simulink model "PID_PMSM_Version_final"  (R2022b)
settings: Solver=VariableStepAuto  StartTime=0.0  StopTime=6  RelTol=1e-3
InitFcn:
  | %% PMSM parameter initialization
  | % switching freq, sample time
  | Ts = 5e-6;          % Fundamental sample time
  | Fsw = 5e3;          % Switching frequency (Hz)
  | Tsw =  1/Fsw ;      %1/Fsw ; Time Switching
  | Tsc = 5e-6  ;       %1/fc;  % Control loop sample time
  | fc = 1/Tsc;         % Control loop frequency (Hz)
  | % ================================================
  | 
  | % PMSM parameters
  | Ld = 0.006365;          % Stator inductance
  | Lq = 0.006365 ;
  | Rs = 1.6;               % Stator Resistance
  | Lambda_m = 0.1852;      % Permanent Flux linkage
  | Polepairs = 4; N = 4;   % Number of pole pairs
  | J = 0.0001854;          % Moment of inertia
  | B = 5.39e-5;            % Viscous coefficient
  | 
  | Vnorm = 300;            % Vdc voltage (DC-bus)
  | Vbat = 350 ;           % Battery voltage (supply the inverter)
undefined symbols (not defined in the file or in its folder): sigbuilder_block
libraries: spsIGBTDiodeLib x6, slpidlib x3, spsDCVoltageSourceLib x1, spsGroundLib x1, spsPermanentMagnetSynchronousMachineLib x1, spsThreePhaseVIMeasurementLib x1, spsCurrentMeasurementLib x1, spsVoltageMeasurementLib x1, eeTransforms x1, simulink_extras x1, spspowerguiLib x1
settings Model: Creator=M. Yahia  LastModifiedBy=muham

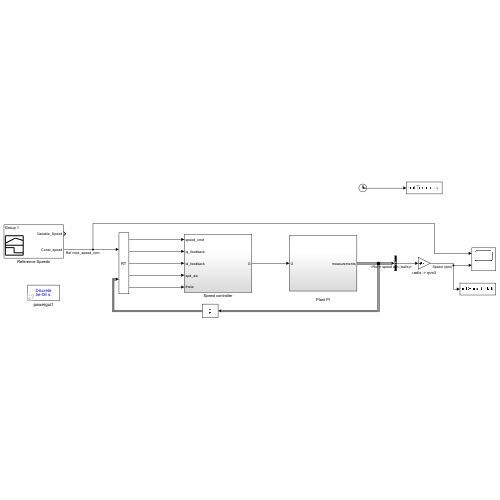
[thumbnail: Simulink's stored preview of the top-level diagram]
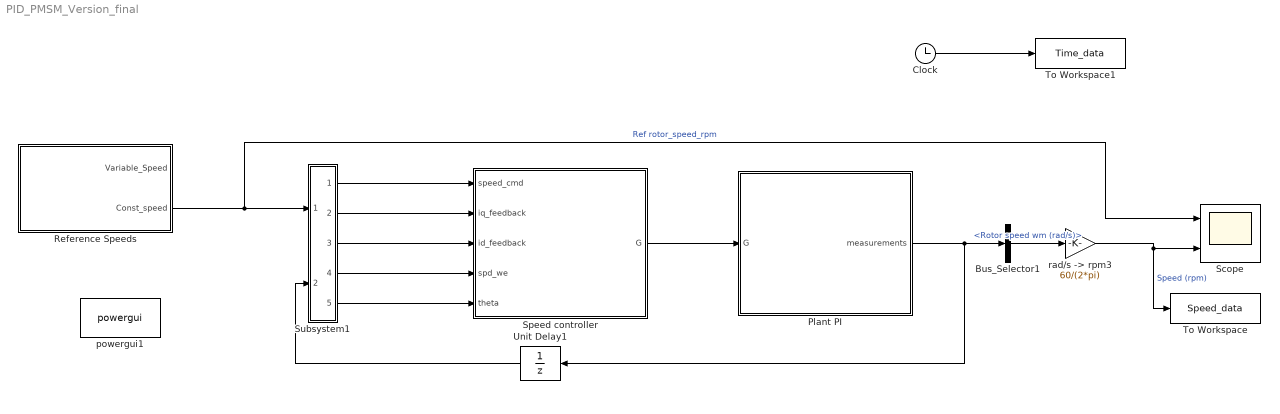
== system PID_PMSM_Version_final ==
  " Plant PI" : Subsystem
  Bus_Selector1 : BusSelector  OutputSignals=Rotor speed wm (rad/s)
  Clock : Clock
  Reference Speeds : Subsystem  Tag=STV Subsys  LoadFcn=sigbuilder_block('load');  StartFcn=sigbuilder_block('start');  StopFcn=sigbuilder_block('stop');  ClipboardFcn=sigbuilder_block('clipboard');  mask(Sigbuilder block){tuvar=[0:10]}
      mask help: Simulink:masks:SigbuilderBlock_MD
      mask init:
      | if ~strcmp(get_param(bdroot(gcbh),'SimulationStatus'),'stopped') tuvar = sigbuilder_block('maskInit'); end
      settings: CopyFcn=sigbuilder_block('copy');  DeleteFcn=sigbuilder_block('delete');  ModelCloseFcn=sigbuilder_block('modelClose');  PreSaveFcn=sigbuilder_block('preSave');  PauseFcn=sigbuilder_block('pause');  ContinueFcn=sigbuilder_block('continue');  NameChangeFcn=sigbuilder_block('namechange');  OpenFcn=sigbuilder_block('open',[34.8 97.5 688.2 385.125 ]);  CloseFcn=sigbuilder_block('close');
      mask Display: plot(0, 0, 100, 100,[2, 2, 32, 32, 2], [68, 8, 8, 68, 68],[32, 2], [38, 38], [32, 19, 2],[53, 60, 44], [32, 17, 17, 2],[16, 16, 31, 31]);txt = getActiveGroup(gcbh);text(2, 100, txt,'verticalAlignment', 'top');
  Scope : Scope  NumInputPorts=2
  Speed controller : Subsystem
  Subsystem1 : Subsystem
      mask Display: fprintf('RT')
  To Workspace : ToWorkspace  VariableName=Speed_data  SaveFormat=Timeseries  SampleTime=-1
  To Workspace1 : ToWorkspace  VariableName=Time_data  SaveFormat=Timeseries  SampleTime=-1
  Unit Delay1 : UnitDelay  SampleTime=-1  HasFrameUpgradeWarning=on
  powergui1 : spspowerguiLib/powergui  SimulationMode=Discrete  SampleTime=Ts  frequency=60  Iterations=50  frequencyindice=0  Pbase=100e6  ErrMax=1e-4  UnitsV=kV  UnitsW=MW  buscounter=0  FunctionMessages=off  echomessages=off  EnableUseOfTLC=off  CurrentSourceSwitches=off  DisableSnubberDevices=off  DisableRonSwitches=off  DisableVfSwitches=off  DisplayEquations=off  AutomaticDiscreteSolvers=off  SolverType=Tustin/Backward Euler (TBE)  Interpol=off  ExternalGateDelay=off  methode=off  Ts=100  x0status=blocks  SPID=on  SwTol=0  HookPort=off  NonlinearTolerance=1e-4  nMaxIteration=100  ContinueOnMaxIteration=off  RestoreLinks=warning  ResistiveCurrentMeasurement=off  Frange=[0:2:500]  Ylog=off  Xlog=on  ShowGrid=off  save=off  variable=ZData  structure=0  ZoomFFT=on  StartTime=0.0  cycles=1  DisplayStyle=1  fundamental=60  FreqAxis=off  MaxFrequency=1000  frequencyindicesteady=1  RmsSteady=1  display=off
  "rad/s -> rpm3" : Gain  Gain=60/(2*pi)
  wires:
  Unit Delay1/1 -> Subsystem1/2(PMSM_Measurements)
  Bus_Selector1/1 -> "rad/s -> rpm3"/1  "<Rotor speed wm (rad/s)>"
  Subsystem1/3(Out3) -> Speed controller/3(id_feedback)
  Speed controller/1(G) -> " Plant PI"/1(G)
  " Plant PI"/1(measurements) -> Bus_Selector1/1, Unit Delay1/1
  Subsystem1/4(Out1) -> Speed controller/4(spd_we)
  Subsystem1/2(Out2) -> Speed controller/2(iq_feedback)
  Subsystem1/5(Out4) -> Speed controller/5(theta)
  Subsystem1/1(Out6) -> Speed controller/1(speed_cmd)
  "rad/s -> rpm3"/1 -> To Workspace/1, Scope/2  "Speed (rpm)"
  Clock/1 -> To Workspace1/1
  Reference Speeds/2(Const_speed) -> Scope/1, Subsystem1/1(speed_cmd)  "Ref rotor_speed_rpm"

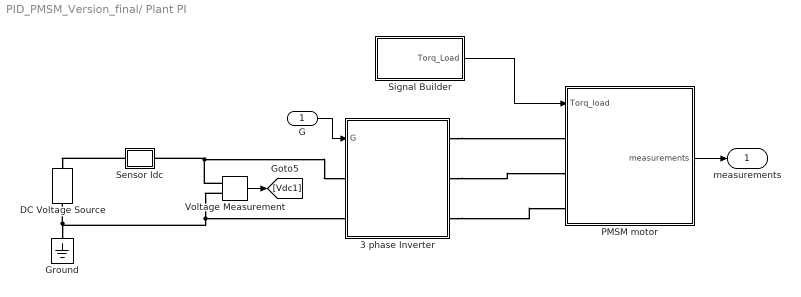
== system PID_PMSM_Version_final/ Plant PI ==
  G : Inport
  3 phase Inverter : Subsystem
  DC Voltage Source : spsDCVoltageSourceLib/DC Voltage Source  Amplitude=Vbat  Measurements=None
  Ground : spsGroundLib/Ground  LConnTagsString=a
  PMSM motor : Subsystem
  Sensor Idc : Subsystem
      mask Display: disp('Idc')
  Signal Builder : Subsystem  Tag=STV Subsys  LoadFcn=sigbuilder_block('load');  StartFcn=sigbuilder_block('start');  StopFcn=sigbuilder_block('stop');  ClipboardFcn=sigbuilder_block('clipboard');  mask(Sigbuilder block){tuvar=[0:10]}
      mask help: Simulink:masks:SigbuilderBlock_MD
      mask init:
      | if ~strcmp(get_param(bdroot(gcbh),'SimulationStatus'),'stopped') tuvar = sigbuilder_block('maskInit'); end
      settings: CopyFcn=sigbuilder_block('copy');  DeleteFcn=sigbuilder_block('delete');  ModelCloseFcn=sigbuilder_block('modelClose');  PreSaveFcn=sigbuilder_block('preSave');  PauseFcn=sigbuilder_block('pause');  ContinueFcn=sigbuilder_block('continue');  NameChangeFcn=sigbuilder_block('namechange');  OpenFcn=sigbuilder_block('open',[354.375 129 543.75 350.625 ]);  CloseFcn=sigbuilder_block('close');
      mask Display: plot(0, 0, 100, 100,[2, 2, 32, 32, 2], [68, 8, 8, 68, 68],[32, 2], [38, 38], [32, 19, 2],[53, 60, 44], [32, 17, 17, 2],[16, 16, 31, 31]);txt = getActiveGroup(gcbh);text(2, 100, txt,'verticalAlignment', 'top');
  Voltage Measurement : spsVoltageMeasurementLib/Voltage Measurement  PhasorSimulation=off  OutputType=Complex  PSBequivalent=0
  measurements : Outport
  wires:
  G/1 -> 3 phase Inverter/1(G)
  Voltage Measurement/1 -> [Vdc1]
  PMSM motor/1(measurements) -> measurements/1
  Signal Builder/1(Torq_Load) -> PMSM motor/1(Torq_load)
  connections:
  Voltage Measurement/LConn2 -- Ground/LConn1 -- DC Voltage Source/LConn1 -- 3 phase Inverter/LConn2
  Voltage Measurement/LConn1 -- Sensor Idc/RConn1 -- 3 phase Inverter/LConn1
  Sensor Idc/LConn1 -- DC Voltage Source/RConn1
  3 phase Inverter/RConn1 -- PMSM motor/LConn1
  3 phase Inverter/RConn2 -- PMSM motor/LConn2
  3 phase Inverter/RConn3 -- PMSM motor/LConn3

== system PID_PMSM_Version_final/Reference Speeds ==
  Demux : Demux  Tag=STV Demux  Outputs=2
      settings: DisplayOption=none
  FromWs : FromWorkspace  Tag=STV FromWs  VariableName=tuvar
      SigBuilderData=|
      | common.afterFinalStr = 'Extrapolate'
      | common.sampleTime = 0
      | dataSet.timeRange = [0 6]
      | dataSet.name = 'Group 1'
      | sbobj.Groups.Name = 'Group 1'
      | sbobj.Groups.Signals(1).Name = 'Variable_Speed'
      | sbobj.Groups.Signals(1).XData = [0 0.2 0.5 0.7 0.8 1.2 1.5 2.2 2.2 2.8 3 3.5 4 4.5 4.5 5.5 6]
      | sbobj.Groups.Signals(1).YData = [40 40 500 200 1000 1000 450 1500 2000 2000 600 600 2000 2000 1000 200 20]
      | sbobj.Groups.Signals(2).Name = 'Const_speed'
      | sbobj.Groups.Signals(2).XData = [0 6]
      | sbobj.Groups.Signals(2).YData = [1000 1000]
      | sbobj.Groups.TimeRange = [0 6]
  Variable_Speed : Outport  Tag=STV Outport  VectorParamsAs1DForOutWhenUnconnected=off
  Const_speed : Outport  Tag=STV Outport  Port=2
  wires:
  Demux/1 -> Variable_Speed/1
  FromWs/1 -> Demux/1
  Demux/2 -> Const_speed/1

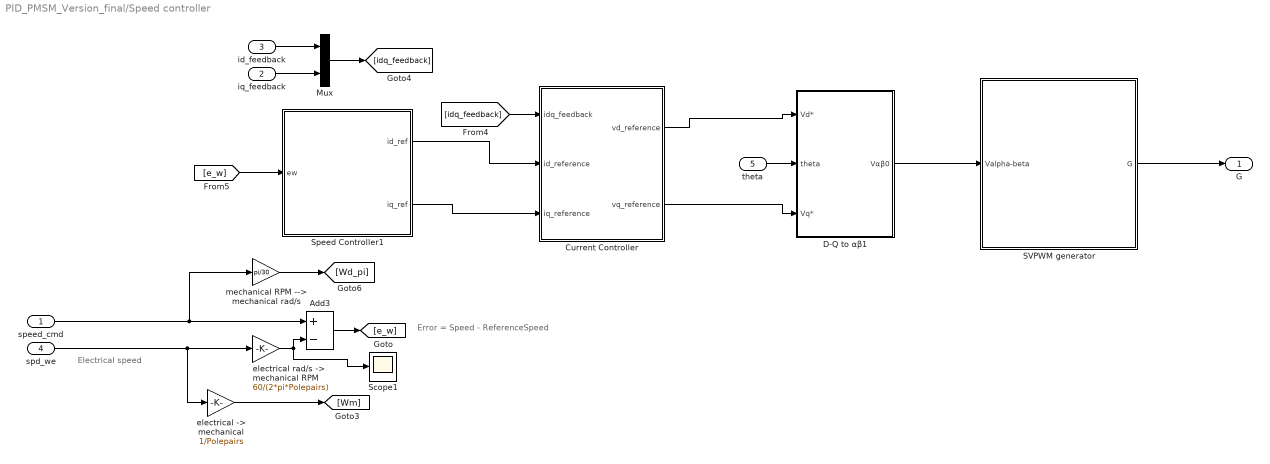
== system PID_PMSM_Version_final/Speed controller ==
  note: Error = Speed - ReferenceSpeed
  note: Electrical speed
  speed_cmd : Inport
  iq_feedback : Inport  Port=2  SampleTime=1e-4
  id_feedback : Inport  Port=3  SampleTime=1e-4
  spd_we : Inport  Port=4
  theta : Inport  Port=5  SampleTime=1e-4
  Add3 : Sum  Inputs=+-
  Current Controller : Subsystem
  D-Q to αβ1 : Subsystem
  Mux : Mux  Inputs=2
  SVPWM generator : Subsystem
  Scope1 : Scope
  Speed Controller1 : Subsystem
  "electrical -> mechanical" : Gain  Gain=1/Polepairs
  "electrical rad/s -> mechanical RPM" : Gain  Gain=60/(2*pi*Polepairs)
  "mechanical RPM --> mechanical rad/s " : Gain  Gain=pi/30
  G : Outport
  wires:
  Speed Controller1/2(iq_ref) -> Current Controller/3(iq_reference)
  Speed Controller1/1(id_ref) -> Current Controller/2(id_reference)
  id_feedback/1 -> Mux/1
  iq_feedback/1 -> Mux/2
  theta/1 -> D-Q to αβ1/2(theta)
  Add3/1 -> [e_w]
  "electrical -> mechanical"/1 -> [Wm]
  spd_we/1 -> "electrical -> mechanical"/1, "electrical rad/s -> mechanical RPM"/1
  "electrical rad/s -> mechanical RPM"/1 -> Scope1/1, Add3/2
  speed_cmd/1 -> "mechanical RPM --> mechanical rad/s "/1, Add3/1
  "mechanical RPM --> mechanical rad/s "/1 -> [Wd_pi]
  Mux/1 -> [idq_feedback]
  [idq_feedback] -> Current Controller/1(idq_feedback)
  [e_w] -> Speed Controller1/1(ew)
  Current Controller/1(vd_reference) -> D-Q to αβ1/1(Vd*)
  Current Controller/2(vq_reference) -> D-Q to αβ1/3(Vq*)
  SVPWM generator/1(G) -> G/1
  D-Q to αβ1/1("Vαβ0 ") -> SVPWM generator/1(Valpha-beta)

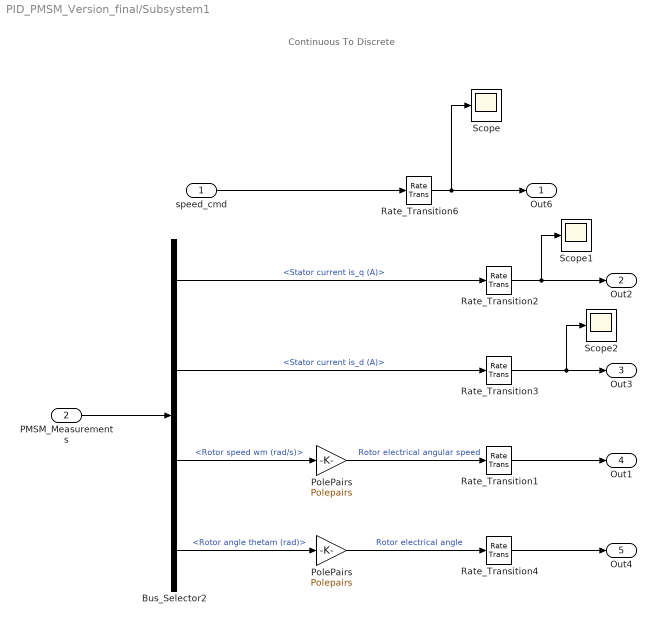
== system PID_PMSM_Version_final/Subsystem1 ==
  note: Continuous To Discrete
  speed_cmd : Inport
  PMSM_Measurements : Inport  Port=2
  Bus_Selector2 : BusSelector  OutputSignals=Stator current is_q (A),Stator current is_d (A),Rotor speed wm (rad/s),Rotor angle thetam (rad)
  PolePairs : Gain  Gain=Polepairs
  "PolePairs " : Gain  Gain=Polepairs
  Rate_Transition{1..4,6} (5 alike) : RateTransition  Integrity=off  Deterministic=off
  Scope : Scope
  Scope1 : Scope
  Scope2 : Scope
  Out6 : Outport  VectorParamsAs1DForOutWhenUnconnected=off
  Out2 : Outport  Port=2  VectorParamsAs1DForOutWhenUnconnected=off
  Out3 : Outport  Port=3  VectorParamsAs1DForOutWhenUnconnected=off
  Out1 : Outport  Port=4  VectorParamsAs1DForOutWhenUnconnected=off
  Out4 : Outport  Port=5  VectorParamsAs1DForOutWhenUnconnected=off
  wires:
  Rate_Transition4/1 -> Out4/1
  Bus_Selector2/2 -> Rate_Transition3/1  "<Stator current is_d (A)>"
  speed_cmd/1 -> Rate_Transition6/1
  Bus_Selector2/1 -> Rate_Transition2/1  "<Stator current is_q (A)>"
  Bus_Selector2/4 -> PolePairs/1  "<Rotor angle thetam (rad)>"
  PMSM_Measurements/1 -> Bus_Selector2/1
  PolePairs/1 -> Rate_Transition4/1  "Rotor electrical angle"
  Rate_Transition6/1 -> Out6/1, Scope/1
  Rate_Transition2/1 -> Scope1/1, Out2/1
  Rate_Transition3/1 -> Scope2/1, Out3/1
  Rate_Transition1/1 -> Out1/1
  Bus_Selector2/3 -> "PolePairs "/1  "<Rotor speed wm (rad/s)>"
  "PolePairs "/1 -> Rate_Transition1/1  "Rotor electrical angular speed"

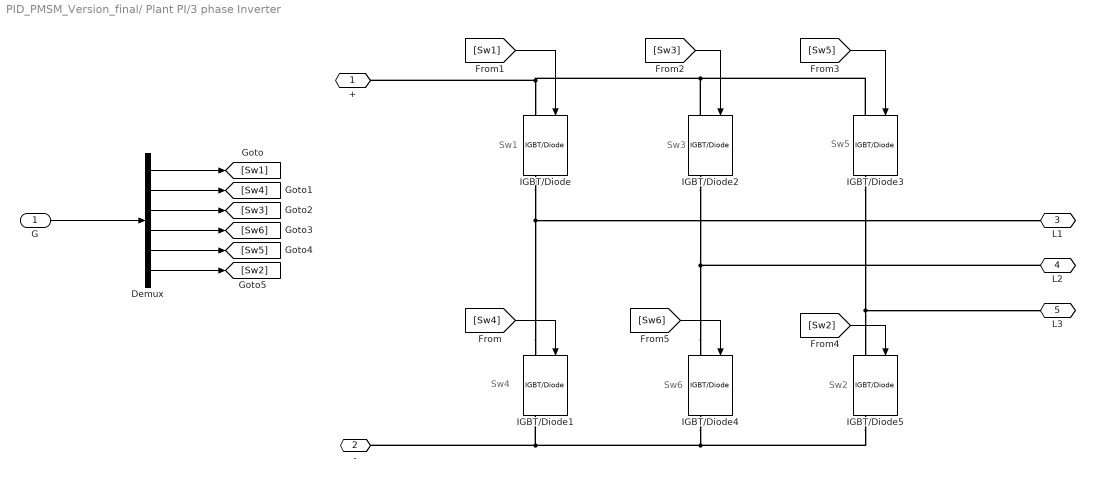
== system PID_PMSM_Version_final/ Plant PI/3 phase Inverter ==
  note: Sw1
  note: Sw4
  note: Sw3
  note: Sw5
  note: Sw2
  note: Sw6
  G : Inport
  Demux : Demux  Outputs=6
  IGBT/Diode{,1..5} (6 alike) : spsIGBTDiodeLib/IGBT//Diode  Ron=1e-3  Rs=1e5  Cs=inf  Measurements=on
  + : PMIOPort  Tag=PMCPort  Side=Left
  - : PMIOPort  Tag=PMCPort  Port=2  Side=Left
  L1 : PMIOPort  Tag=PMCPort  Port=3  Side=Right
  L2 : PMIOPort  Tag=PMCPort  Port=4  Side=Right
  L3 : PMIOPort  Tag=PMCPort  Port=5  Side=Right
  wires:
  G/1 -> Demux/1
  Demux/1 -> [Sw1]
  Demux/2 -> [Sw4]
  Demux/4 -> [Sw6]
  Demux/3 -> [Sw3]
  Demux/5 -> [Sw5]
  Demux/6 -> [Sw2]
  [Sw1] -> IGBT/Diode/1
  [Sw5] -> IGBT/Diode3/1
  [Sw6] -> IGBT/Diode4/1
  [Sw4] -> IGBT/Diode1/1
  [Sw3] -> IGBT/Diode2/1
  [Sw2] -> IGBT/Diode5/1
  connections:
  IGBT/Diode1/LConn1 -- L1/RConn1 -- IGBT/Diode/RConn1
  IGBT/Diode3/RConn1 -- IGBT/Diode5/LConn1 -- L3/RConn1
  IGBT/Diode4/LConn1 -- L2/RConn1 -- IGBT/Diode2/RConn1
  IGBT/Diode3/LConn1 -- IGBT/Diode2/LConn1 -- IGBT/Diode/LConn1 -- +/RConn1
  IGBT/Diode4/RConn1 -- -/RConn1 -- IGBT/Diode1/RConn1 -- IGBT/Diode5/RConn1

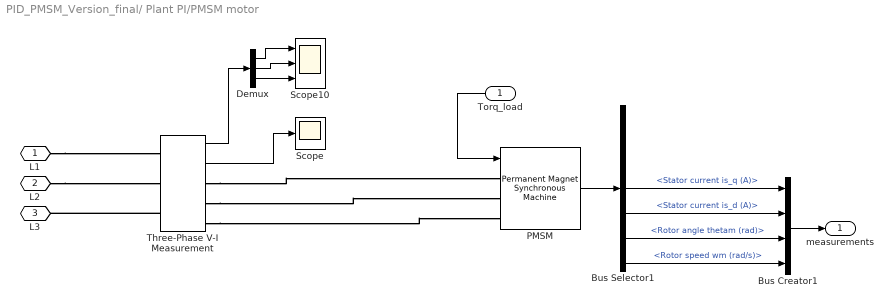
== system PID_PMSM_Version_final/ Plant PI/PMSM motor ==
  Torq_load : Inport
  Bus Creator1 : BusCreator  Inputs=4
  Bus Selector1 : BusSelector  OutputSignals=Stator current is_a (A),Stator current is_b (A),Stator current is_c (A),Stator current is_q (A),Stator current is_d (A),Rotor angle thetam (rad),Rotor speed wm (rad/s)
  Demux : Demux  Outputs=3
  PMSM : spsPermanentMagnetSynchronousMachineLib/Permanent Magnet Synchronous Machine  NbPhases=3  FluxDistribution=Sinusoidal  RotorType=Round  MechanicalLoad=Torque Tm  PresetModel=No  ShowDetailedParameters=on  MeasurementBus=off  Resistance=Rs  Inductance=8.5e-3  dqInductances=[Ld,Lq]  La=Ld  MachineConstant=Flux linkage established by magnets (V.s)  Flux=Lambda_m  VoltageCst=134.3663  TorqueCst=1.1112  Flat=120  Mechanical=[J B Polepairs 0]  PolePairs=2  InitialConditions=[0,0, 0,0]  InitialConditions5ph=[0 0 0 0 0 0]  RefAngle=Aligned with phase A axis (original Park)  IterativeDiscreteModel=Trapezoidal robust  TsBlock=Ts  TsPowergui=0
  Scope : Scope
  Scope10 : Scope  NumInputPorts=3
  Three-Phase V-I Measurement : spsThreePhaseVIMeasurementLib/Three-Phase V-I Measurement  VoltageMeasurement=phase-to-phase  SetLabelV=off  LabelV=Vabc  Vpu=off  VpuLL=off  CurrentMeasurement=yes  SetLabelI=off  LabelI=Iabc  Ipu=off  Pbase=100e6  Vbase=500e3  OutputType=Complex  PhasorSimulation=off  PSBequivalent=0
  L1 : PMIOPort  Side=Left
  L2 : PMIOPort  Port=2  Side=Left
  L3 : PMIOPort  Port=3  Side=Left
  measurements : Outport  VectorParamsAs1DForOutWhenUnconnected=off
  wires:
  Torq_load/1 -> PMSM/1
  Bus Selector1/4 -> Bus Creator1/1  "<Stator current is_q (A)>"
  Bus Selector1/5 -> Bus Creator1/2  "<Stator current is_d (A)>"
  Bus Creator1/1 -> measurements/1
  Bus Selector1/7 -> Bus Creator1/4  "<Rotor speed wm (rad/s)>"
  Bus Selector1/6 -> Bus Creator1/3  "<Rotor angle thetam (rad)>"
  PMSM/1 -> Bus Selector1/1
  Three-Phase V-I Measurement/2 -> Scope/1
  Demux/3 -> Scope10/3
  Demux/1 -> Scope10/1
  Demux/2 -> Scope10/2
  Three-Phase V-I Measurement/1 -> Demux/1
  connections:
  Three-Phase V-I Measurement/RConn2 -- PMSM/LConn2
  Three-Phase V-I Measurement/RConn3 -- PMSM/LConn3
  Three-Phase V-I Measurement/RConn1 -- PMSM/LConn1
  L1/RConn1 -- Three-Phase V-I Measurement/LConn1
  L2/RConn1 -- Three-Phase V-I Measurement/LConn2
  Three-Phase V-I Measurement/LConn3 -- L3/RConn1

== system PID_PMSM_Version_final/ Plant PI/Sensor Idc ==
  Current Measurement : spsCurrentMeasurementLib/Current Measurement  PhasorSimulation=off  OutputType=Complex  PSBequivalent=0
  + : PMIOPort  Side=Left
  - : PMIOPort  Port=2  Side=Right
  wires:
  Current Measurement/1 -> [Idc1]
  connections:
  +/RConn1 -- Current Measurement/LConn1
  -/RConn1 -- Current Measurement/RConn1

== system PID_PMSM_Version_final/ Plant PI/Signal Builder ==
  Demux : Demux  Tag=STV Demux  Outputs=1
      settings: DisplayOption=none
  FromWs : FromWorkspace  Tag=STV FromWs  VariableName=tuvar
      SigBuilderData=|
      | common.afterFinalStr = 'Extrapolate'
      | common.sampleTime = 0
      | dataSet.timeRange = [0 6]
      | dataSet.name = 'Group 1'
      | sbobj.Groups.Name = 'Group 1'
      | sbobj.Groups.Signals.Name = 'Torq_Load'
      | sbobj.Groups.Signals.XData = [0 0.5 1 1.5 2 2.5 3 3 3.5 4 4 5 5.5 6]
      | sbobj.Groups.Signals.YData = [0 0 0 0 0 0 0 1 1 1 0 0 0 0]
      | sbobj.Groups.TimeRange = [0 6]
  Torq_Load : Outport  Tag=STV Outport
  wires:
  Demux/1 -> Torq_Load/1
  FromWs/1 -> Demux/1

== system PID_PMSM_Version_final/Speed controller/Current Controller ==
  idq_feedback : Inport  SampleTime=1e-4
  id_reference : Inport  Port=2  SampleTime=1e-4
  iq_reference : Inport  Port=3  SampleTime=1e-4
  Demux : Demux  Outputs=2
  PID Controller : slpidlib/PID Controller  Controller=PI  Form=Parallel  TimeDomain=Discrete-time  UseExternalTs=off  SampleTime=-1  IntegratorMethod=Forward Euler  FilterMethod=Forward Euler  ControllerParametersSource=internal  P=86  I=13  UseKiTs=off  D=0  N=100  UseFilter=on  TunerSelectOption=Transfer Function Based (PID Tuner App)  InitialConditionSource=internal  InitialConditionForIntegrator=0  InitialConditionForFilter=0  DifferentiatorICPrevScaledInput=0  ExternalReset=none  TrackingMode=off  Kt=1  LimitOutput=off  SatLimitsSource=internal  UpperSaturationLimit=inf  LowerSaturationLimit=-inf  LinearizeAsGain=on  AntiWindupMode=none  Kb=1  LimitIntegrator=off  UpperIntegratorSaturationLimit=inf  LowerIntegratorSaturationLimit=-inf  POutMin=[]  POutMax=[]  IOutMin=[]  IOutMax=[]  DOutMin=[]  DOutMax=[]  NOutMin=[]  NOutMax=[]  SumOutMin=[]  SumOutMax=[]  SaturationOutMin=[]  SaturationOutMax=[]  PParamMin=[]  PParamMax=[]  IParamMin=[]  IParamMax=[]  DParamMin=[]  DParamMax=[]  NParamMin=[]  NParamMax=[]  KbParamMin=[]  KbParamMax=[]  KtParamMin=[]  KtParamMax=[]  KbOutMin=[]  KbOutMax=[]  KtOutMin=[]  KtOutMax=[]  IntegratorOutMin=[]  IntegratorOutMax=[]  FilterOutMin=[]  FilterOutMax=[]  SumI1OutMin=[]  SumI1OutMax=[]  SumI2OutMin=[]  SumI2OutMax=[]  SumI3OutMin=[]  SumI3OutMax=[]  SumI4OutMin=[]  SumI4OutMax=[]  SumDOutMin=[]  SumDOutMax=[]  DifferentiatorOutMin=[]  DifferentiatorOutMax=[]  FilterDiffOutCoefMin=[]  FilterDiffOutCoefMax=[]  ReciprocalOutMin=[]  ReciprocalOutMax=[]  SumDenOutMin=[]  SumDenOutMax=[]  SumNumOutMin=[]  SumNumOutMax=[]  DivideOutMin=[]  DivideOutMax=[]  UdiffTsProdOutMin=[]  UdiffTsProdOutMax=[]  NTsProdOutMin=[]  NTsProdOutMax=[]  UintegralTsProdOutMin=[]  UintegralTsProdOutMax=[]  UngainTsProdOutMin=[]  UngainTsProdOutMax=[]  ClampingZeroOutDataTypeStr=Inherit: Inherit via back propagation  ClampingZeroOutMin=[]  ClampingZeroOutMax=[]  FilterDenConstantOutDataTypeStr=Inherit: Inherit via back propagation  FilterDenConstantOutMin=[]  FilterDenConstantOutMax=[]  PCopyOutDataTypeStr=Inherit: Inherit via back propagation  PCopyOutMin=[]  PCopyOutMax=[]  NCopyOutDataTypeStr=Inherit: Inherit via back propagation  NCopyOutMin=[]  NCopyOutMax=[]  IntegratorContinuousStateAttributes=''  IntegratorStateMustResolveToSignalObject=off  IntegratorRTWStateStorageClass=Auto  FilterContinuousStateAttributes=''  FilterStateMustResolveToSignalObject=off  FilterRTWStateStorageClass=Auto  ParallelPVariant=InternalParameters  IdealPVariant=Disabled  IVariant=InternalParameters  DVariant=Disabled  IntegratorVariant=Discrete  SatVariant=Disabled  AWVariant=Passthrough  PCopyVariant=Disabled  TRVariant=Disabled  FdbkBlocksVariant=Forward  IdealPFdbkVariant=Disabled  SatFdbkVariant=Disabled  DerivativeFilterVariant=Disabled  NVariant=Disabled  NCopyVariant=Disabled_SignalSpec  FilterICVariant=Disabled  IntegratorICVariant=InternalICs  ExternalResetVariant=Disabled  TRSumVariant=Passthrough  SumFdbkVariant=Disabled  SumVariant=Sum_PI  TsampFilterVariant=InternalTs  TsampNgainVariant=Passthrough  TsampIntegralVariant=Passthrough  ExternalSaturationOutDataTypeStr=Inherit: Same as second input
  PID Controller1 : slpidlib/PID Controller  Controller=PI  Form=Parallel  TimeDomain=Discrete-time  UseExternalTs=off  SampleTime=-1  IntegratorMethod=Forward Euler  FilterMethod=Forward Euler  ControllerParametersSource=internal  P=86  I=13  UseKiTs=off  D=0  N=100  UseFilter=on  TunerSelectOption=Transfer Function Based (PID Tuner App)  InitialConditionSource=internal  InitialConditionForIntegrator=0  InitialConditionForFilter=0  DifferentiatorICPrevScaledInput=0  ExternalReset=none  TrackingMode=off  Kt=1  LimitOutput=off  SatLimitsSource=internal  UpperSaturationLimit=inf  LowerSaturationLimit=-inf  LinearizeAsGain=on  AntiWindupMode=none  Kb=1  LimitIntegrator=off  UpperIntegratorSaturationLimit=inf  LowerIntegratorSaturationLimit=-inf  POutMin=[]  POutMax=[]  IOutMin=[]  IOutMax=[]  DOutMin=[]  DOutMax=[]  NOutMin=[]  NOutMax=[]  SumOutMin=[]  SumOutMax=[]  SaturationOutMin=[]  SaturationOutMax=[]  PParamMin=[]  PParamMax=[]  IParamMin=[]  IParamMax=[]  DParamMin=[]  DParamMax=[]  NParamMin=[]  NParamMax=[]  KbParamMin=[]  KbParamMax=[]  KtParamMin=[]  KtParamMax=[]  KbOutMin=[]  KbOutMax=[]  KtOutMin=[]  KtOutMax=[]  IntegratorOutMin=[]  IntegratorOutMax=[]  FilterOutMin=[]  FilterOutMax=[]  SumI1OutMin=[]  SumI1OutMax=[]  SumI2OutMin=[]  SumI2OutMax=[]  SumI3OutMin=[]  SumI3OutMax=[]  SumI4OutMin=[]  SumI4OutMax=[]  SumDOutMin=[]  SumDOutMax=[]  DifferentiatorOutMin=[]  DifferentiatorOutMax=[]  FilterDiffOutCoefMin=[]  FilterDiffOutCoefMax=[]  ReciprocalOutMin=[]  ReciprocalOutMax=[]  SumDenOutMin=[]  SumDenOutMax=[]  SumNumOutMin=[]  SumNumOutMax=[]  DivideOutMin=[]  DivideOutMax=[]  UdiffTsProdOutMin=[]  UdiffTsProdOutMax=[]  NTsProdOutMin=[]  NTsProdOutMax=[]  UintegralTsProdOutMin=[]  UintegralTsProdOutMax=[]  UngainTsProdOutMin=[]  UngainTsProdOutMax=[]  ClampingZeroOutDataTypeStr=Inherit: Inherit via back propagation  ClampingZeroOutMin=[]  ClampingZeroOutMax=[]  FilterDenConstantOutDataTypeStr=Inherit: Inherit via back propagation  FilterDenConstantOutMin=[]  FilterDenConstantOutMax=[]  PCopyOutDataTypeStr=Inherit: Inherit via back propagation  PCopyOutMin=[]  PCopyOutMax=[]  NCopyOutDataTypeStr=Inherit: Inherit via back propagation  NCopyOutMin=[]  NCopyOutMax=[]  IntegratorContinuousStateAttributes=''  IntegratorStateMustResolveToSignalObject=off  IntegratorRTWStateStorageClass=Auto  FilterContinuousStateAttributes=''  FilterStateMustResolveToSignalObject=off  FilterRTWStateStorageClass=Auto  ParallelPVariant=InternalParameters  IdealPVariant=Disabled  IVariant=InternalParameters  DVariant=Disabled  IntegratorVariant=Discrete  SatVariant=Disabled  AWVariant=Passthrough  PCopyVariant=Disabled  TRVariant=Disabled  FdbkBlocksVariant=Forward  IdealPFdbkVariant=Disabled  SatFdbkVariant=Disabled  DerivativeFilterVariant=Disabled  NVariant=Disabled  NCopyVariant=Disabled_SignalSpec  FilterICVariant=Disabled  IntegratorICVariant=InternalICs  ExternalResetVariant=Disabled  TRSumVariant=Passthrough  SumFdbkVariant=Disabled  SumVariant=Sum_PI  TsampFilterVariant=InternalTs  TsampNgainVariant=Passthrough  TsampIntegralVariant=Passthrough  ExternalSaturationOutDataTypeStr=Inherit: Same as second input
  Sum : Sum  Inputs=|+-
  Sum1 : Sum  Inputs=|-+
  vd_reference : Outport  SampleTime=1e-4  VectorParamsAs1DForOutWhenUnconnected=off
  vq_reference : Outport  Port=2  SampleTime=1e-4  VectorParamsAs1DForOutWhenUnconnected=off
  wires:
  idq_feedback/1 -> Demux/1
  Sum1/1 -> PID Controller/1
  Sum/1 -> PID Controller1/1
  id_reference/1 -> Sum/1
  iq_reference/1 -> Sum1/2
  Demux/2 -> Sum1/1
  Demux/1 -> Sum/2
  PID Controller1/1 -> vd_reference/1
  PID Controller/1 -> vq_reference/1

== system PID_PMSM_Version_final/Speed controller/D-Q to αβ1 ==
  Vd* : Inport
  theta : Inport  Port=2
  Vq* : Inport  Port=3
  Constant : Constant  Value=0  SampleTime=Ts
  Mux : Mux  Inputs=2
  Mux1 : Mux  Inputs=2
  Park to Clarke Angle Transform : eeTransforms/Park to Clarke Angle Transform  AxisAlignment=Q-axis
  "Vαβ0 " : Outport  VectorParamsAs1DForOutWhenUnconnected=off
  wires:
  Vd*/1 -> Mux/1  "Vd*"
  Mux/1 -> Mux1/1  "Vdq*"
  Mux1/1 -> Park to Clarke Angle Transform/1
  Constant/1 -> Mux1/2
  theta/1 -> Park to Clarke Angle Transform/2
  Park to Clarke Angle Transform/1 -> "Vαβ0 "/1
  Vq*/1 -> Mux/2  "Vq*"

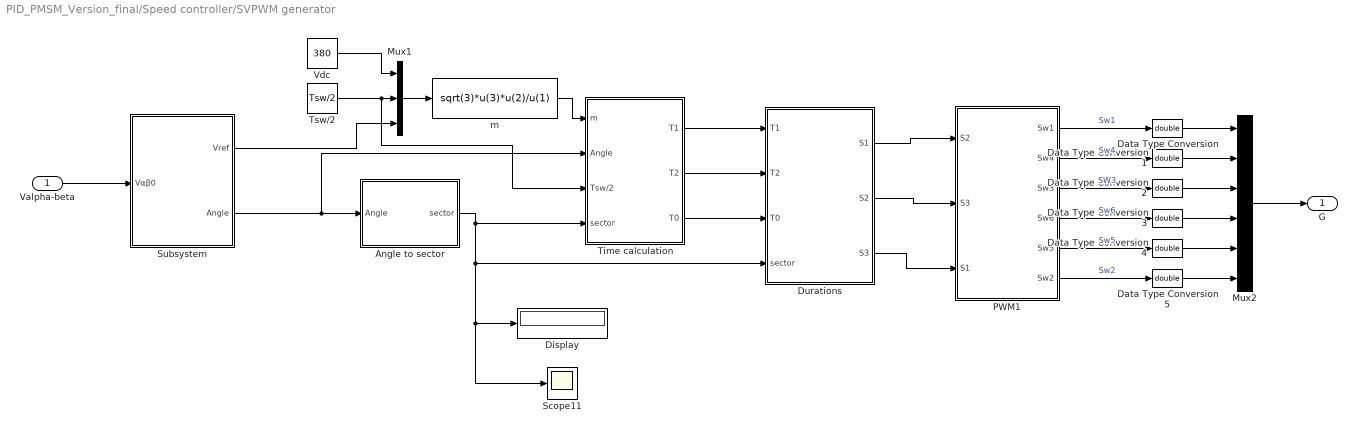
== system PID_PMSM_Version_final/Speed controller/SVPWM generator ==
  Valpha-beta : Inport
  Angle to sector : Subsystem
  Data Type Conversion{,1..5} (6 alike) : DataTypeConversion  OutDataTypeStr=double  SaturateOnIntegerOverflow=off  RndMeth=Floor
  Display : Display
  Durations : Subsystem
  Mux1 : Mux  Inputs=3
  Mux2 : Mux  Inputs=6
  PWM1 : Subsystem
  Scope11 : Scope
  Subsystem : Subsystem
  Time calculation : Subsystem
  Tsw/2 : Constant  Value=Tsw/2
  Vdc : Constant  Value=380
  m : Fcn  Expr=sqrt(3)*u(3)*u(2)/u(1)
  G : Outport
  wires:
  Durations/3(S3) -> PWM1/3(S1)
  Data Type Conversion/1 -> Mux2/1
  Tsw/2/1 -> Time calculation/3(Tsw/2), Mux1/2
  Time calculation/1(T1) -> Durations/1(T1)
  Data Type Conversion5/1 -> Mux2/6
  Data Type Conversion2/1 -> Mux2/3
  Time calculation/3(T0) -> Durations/3(T0)
  PWM1/2(Sw4) -> Data Type Conversion1/1  "Sw4"
  PWM1/3(Sw3) -> Data Type Conversion2/1  "SW3"
  Angle to sector/1(sector) -> Durations/4(sector), Scope11/1, Display/1, Time calculation/4(sector)
  PWM1/4(Sw6) -> Data Type Conversion3/1  "Sw6"
  Vdc/1 -> Mux1/1
  PWM1/6(Sw2) -> Data Type Conversion5/1  "Sw2"
  PWM1/5(Sw5) -> Data Type Conversion4/1  "Sw5"
  m/1 -> Time calculation/1(m)
  Subsystem/2(Angle) -> Angle to sector/1(Angle), Time calculation/2(Angle)
  Mux2/1 -> G/1
  Time calculation/2(T2) -> Durations/2(T2)
  PWM1/1(Sw1) -> Data Type Conversion/1  "Sw1"
  Mux1/1 -> m/1
  Valpha-beta/1 -> Subsystem/1("Vαβ0 ")
  Subsystem/1(Vref) -> Mux1/3
  Data Type Conversion3/1 -> Mux2/4
  Data Type Conversion4/1 -> Mux2/5
  Data Type Conversion1/1 -> Mux2/2
  Durations/2(S2) -> PWM1/2(S3)
  Durations/1(S1) -> PWM1/1(S2)

== system PID_PMSM_Version_final/Speed controller/Speed Controller1 ==
  ew : Inport  SampleTime=1e-3
  Constant : Constant  Value=0
  Constant1 : Constant  Value=Lambda_m*Polepairs
  Divide : Product  Inputs=*/
  Gain : Gain  Gain=3/2
  PID Controller1 : slpidlib/PID Controller  Controller=PI  Form=Parallel  TimeDomain=Discrete-time  UseExternalTs=off  SampleTime=-1  IntegratorMethod=Forward Euler  FilterMethod=Forward Euler  ControllerParametersSource=internal  P=0.02  I=1  UseKiTs=off  D=0  N=100  UseFilter=on  TunerSelectOption=Transfer Function Based (PID Tuner App)  InitialConditionSource=internal  InitialConditionForIntegrator=0  InitialConditionForFilter=0  DifferentiatorICPrevScaledInput=0  ExternalReset=none  TrackingMode=off  Kt=1  LimitOutput=off  SatLimitsSource=internal  UpperSaturationLimit=inf  LowerSaturationLimit=-inf  LinearizeAsGain=on  AntiWindupMode=none  Kb=1  LimitIntegrator=off  UpperIntegratorSaturationLimit=inf  LowerIntegratorSaturationLimit=-inf  POutMin=[]  POutMax=[]  IOutMin=[]  IOutMax=[]  DOutMin=[]  DOutMax=[]  NOutMin=[]  NOutMax=[]  SumOutMin=[]  SumOutMax=[]  SaturationOutMin=[]  SaturationOutMax=[]  PParamMin=[]  PParamMax=[]  IParamMin=[]  IParamMax=[]  DParamMin=[]  DParamMax=[]  NParamMin=[]  NParamMax=[]  KbParamMin=[]  KbParamMax=[]  KtParamMin=[]  KtParamMax=[]  KbOutMin=[]  KbOutMax=[]  KtOutMin=[]  KtOutMax=[]  IntegratorOutMin=[]  IntegratorOutMax=[]  FilterOutMin=[]  FilterOutMax=[]  SumI1OutMin=[]  SumI1OutMax=[]  SumI2OutMin=[]  SumI2OutMax=[]  SumI3OutMin=[]  SumI3OutMax=[]  SumI4OutMin=[]  SumI4OutMax=[]  SumDOutMin=[]  SumDOutMax=[]  DifferentiatorOutMin=[]  DifferentiatorOutMax=[]  FilterDiffOutCoefMin=[]  FilterDiffOutCoefMax=[]  ReciprocalOutMin=[]  ReciprocalOutMax=[]  SumDenOutMin=[]  SumDenOutMax=[]  SumNumOutMin=[]  SumNumOutMax=[]  DivideOutMin=[]  DivideOutMax=[]  UdiffTsProdOutMin=[]  UdiffTsProdOutMax=[]  NTsProdOutMin=[]  NTsProdOutMax=[]  UintegralTsProdOutMin=[]  UintegralTsProdOutMax=[]  UngainTsProdOutMin=[]  UngainTsProdOutMax=[]  ClampingZeroOutDataTypeStr=Inherit: Inherit via back propagation  ClampingZeroOutMin=[]  ClampingZeroOutMax=[]  FilterDenConstantOutDataTypeStr=Inherit: Inherit via back propagation  FilterDenConstantOutMin=[]  FilterDenConstantOutMax=[]  PCopyOutDataTypeStr=Inherit: Inherit via back propagation  PCopyOutMin=[]  PCopyOutMax=[]  NCopyOutDataTypeStr=Inherit: Inherit via back propagation  NCopyOutMin=[]  NCopyOutMax=[]  IntegratorContinuousStateAttributes=''  IntegratorStateMustResolveToSignalObject=off  IntegratorRTWStateStorageClass=Auto  FilterContinuousStateAttributes=''  FilterStateMustResolveToSignalObject=off  FilterRTWStateStorageClass=Auto  ParallelPVariant=InternalParameters  IdealPVariant=Disabled  IVariant=InternalParameters  DVariant=Disabled  IntegratorVariant=Discrete  SatVariant=Disabled  AWVariant=Passthrough  PCopyVariant=Disabled  TRVariant=Disabled  FdbkBlocksVariant=Forward  IdealPFdbkVariant=Disabled  SatFdbkVariant=Disabled  DerivativeFilterVariant=Disabled  NVariant=Disabled  NCopyVariant=Disabled_SignalSpec  FilterICVariant=Disabled  IntegratorICVariant=InternalICs  ExternalResetVariant=Disabled  TRSumVariant=Passthrough  SumFdbkVariant=Disabled  SumVariant=Sum_PI  TsampFilterVariant=InternalTs  TsampNgainVariant=Passthrough  TsampIntegralVariant=Passthrough  ExternalSaturationOutDataTypeStr=Inherit: Same as second input
  id_ref : Outport  VectorParamsAs1DForOutWhenUnconnected=off
  iq_ref : Outport  Port=2  VectorParamsAs1DForOutWhenUnconnected=off
  wires:
  Constant/1 -> id_ref/1
  ew/1 -> PID Controller1/1
  PID Controller1/1 -> Divide/1  "Te_ref"
  Constant1/1 -> Gain/1
  Gain/1 -> Divide/2
  Divide/1 -> iq_ref/1

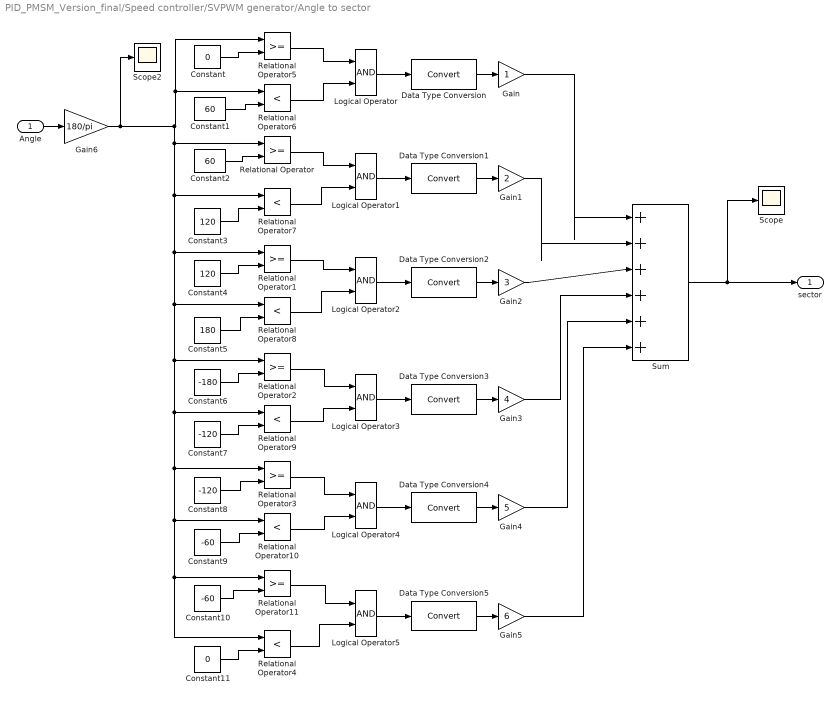
== system PID_PMSM_Version_final/Speed controller/SVPWM generator/Angle to sector ==
  Angle : Inport
  Constant : Constant  Value=0
  Constant1 : Constant  Value=60
  Constant10 : Constant  Value=-60
  Constant11 : Constant  Value=0
  Constant2 : Constant  Value=60
  Constant3 : Constant  Value=120
  Constant4 : Constant  Value=120
  Constant5 : Constant  Value=180
  Constant6 : Constant  Value=-180
  Constant7 : Constant  Value=-120
  Constant8 : Constant  Value=-120
  Constant9 : Constant  Value=-60
  Data Type Conversion{,1..5} (6 alike) : DataTypeConversion  SaturateOnIntegerOverflow=off  RndMeth=Floor
  Gain : Gain
  Gain1 : Gain  Gain=2
  Gain2 : Gain  Gain=3
  Gain3 : Gain  Gain=4
  Gain4 : Gain  Gain=5
  Gain5 : Gain  Gain=6
  Gain6 : Gain  Gain=180/pi
  Logical Operator{,1..5} (6 alike) : Logic  AllPortsSameDT=off  OutDataTypeStr=boolean
  Relational Operator{,1..3,5,11} (6 alike) : RelationalOperator  OutDataTypeStr=boolean  InputSameDT=off
  Relational Operator{4,6..10} (6 alike) : RelationalOperator  Operator=<  OutDataTypeStr=boolean  InputSameDT=off
  Scope : Scope
  Scope2 : Scope
  Sum : Sum  Inputs=|++++++
  sector : Outport
  wires:
  Constant/1 -> Relational Operator5/2
  Constant1/1 -> Relational Operator6/2
  Constant2/1 -> Relational Operator/2
  Constant3/1 -> Relational Operator7/2
  Constant5/1 -> Relational Operator8/2
  Constant6/1 -> Relational Operator2/2
  Constant7/1 -> Relational Operator9/2
  Constant8/1 -> Relational Operator3/2
  Constant9/1 -> Relational Operator10/2
  Constant10/1 -> Relational Operator11/2
  Constant11/1 -> Relational Operator4/2
  Constant4/1 -> Relational Operator1/2
  Relational Operator11/1 -> Logical Operator5/1
  Relational Operator4/1 -> Logical Operator5/2
  Relational Operator3/1 -> Logical Operator4/1
  Relational Operator10/1 -> Logical Operator4/2
  Relational Operator2/1 -> Logical Operator3/1
  Relational Operator9/1 -> Logical Operator3/2
  Relational Operator5/1 -> Logical Operator/1
  Relational Operator6/1 -> Logical Operator/2
  Relational Operator/1 -> Logical Operator1/1
  Relational Operator7/1 -> Logical Operator1/2
  Relational Operator1/1 -> Logical Operator2/1
  Relational Operator8/1 -> Logical Operator2/2
  Gain4/1 -> Sum/5
  Gain3/1 -> Sum/4
  Gain5/1 -> Sum/6
  Gain2/1 -> Sum/3
  Gain1/1 -> Sum/2
  Gain/1 -> Sum/1
  Sum/1 -> Scope/1, sector/1
  Logical Operator/1 -> Data Type Conversion/1
  Data Type Conversion/1 -> Gain/1
  Data Type Conversion1/1 -> Gain1/1
  Logical Operator1/1 -> Data Type Conversion1/1
  Data Type Conversion2/1 -> Gain2/1
  Logical Operator2/1 -> Data Type Conversion2/1
  Data Type Conversion3/1 -> Gain3/1
  Logical Operator3/1 -> Data Type Conversion3/1
  Data Type Conversion4/1 -> Gain4/1
  Logical Operator4/1 -> Data Type Conversion4/1
  Data Type Conversion5/1 -> Gain5/1
  Logical Operator5/1 -> Data Type Conversion5/1
  Angle/1 -> Gain6/1
  Gain6/1 -> Relational Operator/1, Relational Operator7/1, Relational Operator1/1, Relational Operator8/1, Relational Operator2/1, Relational Operator10/1, Relational Operator11/1, Relational Operator4/1, Relational Operator3/1, Relational Operator9/1, Relational Operator6/1, Relational Operator5/1, Scope2/1

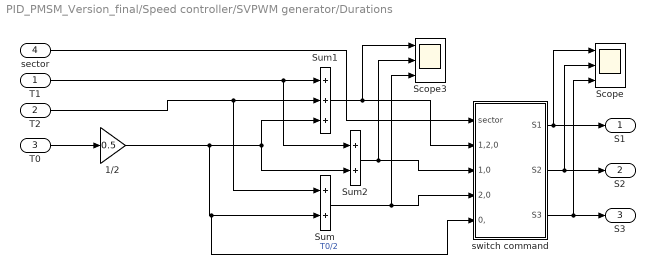
== system PID_PMSM_Version_final/Speed controller/SVPWM generator/Durations ==
  T1 : Inport
  T2 : Inport  Port=2
  T0 : Inport  Port=3
  sector : Inport  Port=4
  1/2 : Gain  Gain=0.5
  Scope : Scope  NumInputPorts=3
  Scope3 : Scope  NumInputPorts=3
  Sum : Sum
  Sum1 : Sum  Inputs=+++
  Sum2 : Sum
  switch command : Subsystem
  S1 : Outport  VectorParamsAs1DForOutWhenUnconnected=off
  S2 : Outport  Port=2  VectorParamsAs1DForOutWhenUnconnected=off
  S3 : Outport  Port=3  VectorParamsAs1DForOutWhenUnconnected=off
  wires:
  Sum/1 -> switch command/4(2,0), Scope3/3
  Sum2/1 -> switch command/3(1,0), Scope3/2
  sector/1 -> switch command/1(sector)
  Sum1/1 -> switch command/2(1,2,0), Scope3/1
  T2/1 -> Sum1/2, Sum/1
  T1/1 -> Sum1/1, Sum2/1
  1/2/1 -> Sum2/2, Sum1/3, Sum/2, switch command/5(0,)  "T0/2"
  switch command/3(S3) -> Scope/3, S3/1
  switch command/2(S2) -> S2/1, Scope/2
  switch command/1(S1) -> S1/1, Scope/1
  T0/1 -> 1/2/1

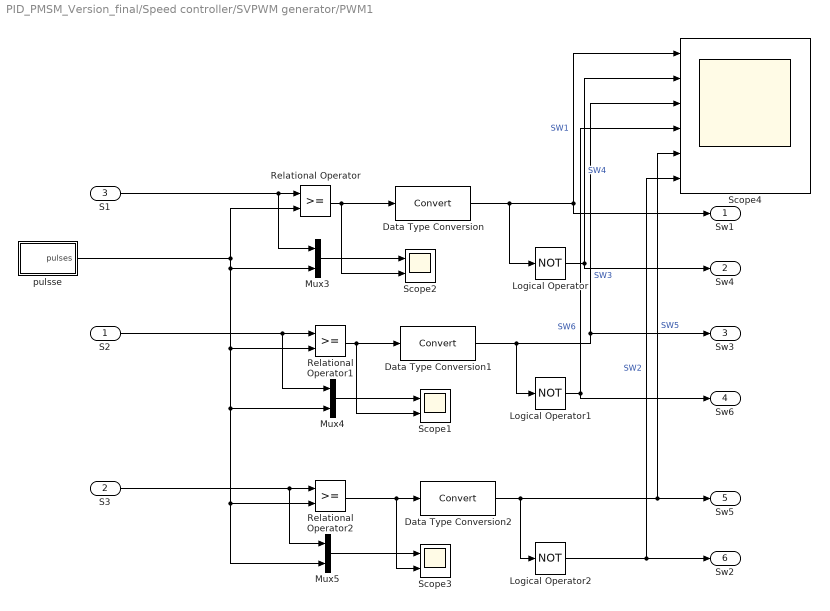
== system PID_PMSM_Version_final/Speed controller/SVPWM generator/PWM1 ==
  S2 : Inport
  S3 : Inport  Port=2
  S1 : Inport  Port=3
  Data Type Conversion : DataTypeConversion  SaturateOnIntegerOverflow=off  RndMeth=Floor
  Data Type Conversion1 : DataTypeConversion  SaturateOnIntegerOverflow=off  RndMeth=Floor
  Data Type Conversion2 : DataTypeConversion  SaturateOnIntegerOverflow=off  RndMeth=Floor
  Logical Operator : Logic  Operator=NOT  AllPortsSameDT=off  OutDataTypeStr=boolean
  Logical Operator1 : Logic  Operator=NOT  AllPortsSameDT=off  OutDataTypeStr=boolean
  Logical Operator2 : Logic  Operator=NOT  AllPortsSameDT=off  OutDataTypeStr=boolean
  Mux3 : Mux  Inputs=2
  Mux4 : Mux  Inputs=2
  Mux5 : Mux  Inputs=2
  Relational Operator : RelationalOperator  OutDataTypeStr=boolean  RndMeth=Ceiling  InputSameDT=off
  Relational Operator1 : RelationalOperator  OutDataTypeStr=boolean  RndMeth=Ceiling  InputSameDT=off
  Relational Operator2 : RelationalOperator  OutDataTypeStr=boolean  RndMeth=Ceiling  InputSameDT=off
  Scope1 : Scope  NumInputPorts=2
  Scope2 : Scope  NumInputPorts=2
  Scope3 : Scope  NumInputPorts=2
  Scope4 : Scope  NumInputPorts=6
  pulsse : Subsystem
  Sw1 : Outport  VectorParamsAs1DForOutWhenUnconnected=off
  Sw4 : Outport  Port=2  VectorParamsAs1DForOutWhenUnconnected=off
  Sw3 : Outport  Port=3  VectorParamsAs1DForOutWhenUnconnected=off
  Sw6 : Outport  Port=4  VectorParamsAs1DForOutWhenUnconnected=off
  Sw5 : Outport  Port=5  VectorParamsAs1DForOutWhenUnconnected=off
  Sw2 : Outport  Port=6  VectorParamsAs1DForOutWhenUnconnected=off
  wires:
  Data Type Conversion2/1 -> Scope4/5, Sw5/1, Logical Operator2/1  "SW5"
  Logical Operator2/1 -> Sw2/1, Scope4/6  "SW2"
  Logical Operator1/1 -> Scope4/4, Sw6/1  "SW6"
  Logical Operator/1 -> Sw4/1, Scope4/2  "SW4"
  pulsse/1(pulses) -> Relational Operator2/2, Mux5/2, Mux4/2, Relational Operator1/2, Mux3/2, Relational Operator/2
  S3/1 -> Relational Operator2/1, Mux5/1
  S2/1 -> Relational Operator1/1, Mux4/1
  S1/1 -> Relational Operator/1, Mux3/1
  Relational Operator/1 -> Scope2/2, Data Type Conversion/1
  Data Type Conversion/1 -> Logical Operator/1, Sw1/1, Scope4/1  "SW1"
  Relational Operator2/1 -> Scope3/2, Data Type Conversion2/1
  Mux5/1 -> Scope3/1
  Data Type Conversion1/1 -> Sw3/1, Scope4/3, Logical Operator1/1  "SW3"
  Relational Operator1/1 -> Scope1/2, Data Type Conversion1/1
  Mux4/1 -> Scope1/1
  Mux3/1 -> Scope2/1

== system PID_PMSM_Version_final/Speed controller/SVPWM generator/Subsystem ==
  "Vαβ0 " : Inport
  Cartesian to Polar1 : simulink_extras/Transformations/Cartesian to Polar
  Demux1 : Demux  Outputs=3
  Display : Display
  Scope1 : Scope
  Zero-Order Hold2 : ZeroOrderHold  SampleTime=Ts
  Zero-Order Hold3 : ZeroOrderHold  SampleTime=Ts
  Vref : Outport
  Angle : Outport  Port=2
  wires:
  Zero-Order Hold3/1 -> Angle/1
  Demux1/1 -> Cartesian to Polar1/1
  Zero-Order Hold2/1 -> Scope1/1, Vref/1
  Demux1/3 -> Display/1
  Cartesian to Polar1/1 -> Zero-Order Hold2/1
  Cartesian to Polar1/2 -> Zero-Order Hold3/1
  Demux1/2 -> Cartesian to Polar1/2
  "Vαβ0 "/1 -> Demux1/1

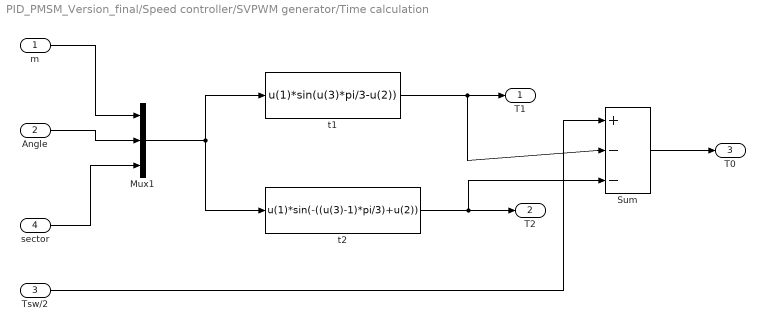
== system PID_PMSM_Version_final/Speed controller/SVPWM generator/Time calculation ==
  m : Inport
  Angle : Inport  Port=2
  Tsw/2 : Inport  Port=3
  sector : Inport  Port=4
  Mux1 : Mux  Inputs=3
  Sum : Sum  Inputs=|+--
  t1 : Fcn  Expr=u(1)*sin(u(3)*pi/3-u(2))
  t2 : Fcn  Expr=u(1)*sin(-((u(3)-1)*pi/3)+u(2))
  T1 : Outport
  T2 : Outport  Port=2
  T0 : Outport  Port=3
  wires:
  m/1 -> Mux1/1
  Angle/1 -> Mux1/2
  sector/1 -> Mux1/3
  Mux1/1 -> t2/1, t1/1
  t1/1 -> Sum/2, T1/1
  t2/1 -> Sum/3, T2/1
  Tsw/2/1 -> Sum/1
  Sum/1 -> T0/1

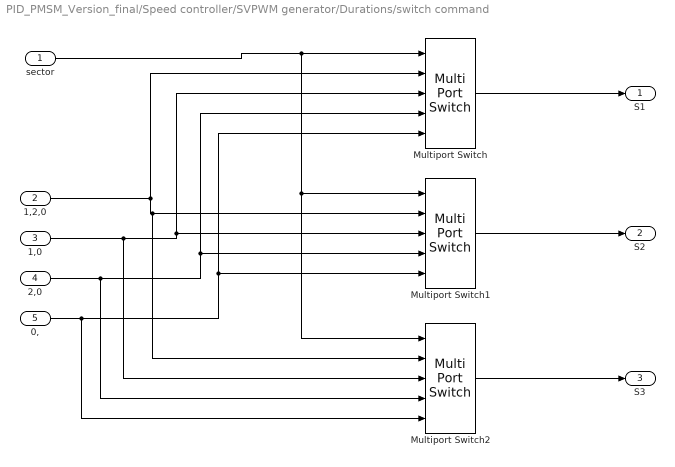
== system PID_PMSM_Version_final/Speed controller/SVPWM generator/Durations/switch command ==
  sector : Inport
  1,2,0 : Inport  Port=2
  1,0 : Inport  Port=3
  2,0 : Inport  Port=4
  0, : Inport  Port=5
  Multiport Switch : MultiPortSwitch  DataPortOrder=Specify indices  DataPortIndices={[1,6],2,5,[3,4]}  DiagnosticForDefault=None  SaturateOnIntegerOverflow=off  InputSameDT=off
  Multiport Switch1 : MultiPortSwitch  DataPortOrder=Specify indices  DataPortIndices={[2,3],4,1,[5,6]}  DiagnosticForDefault=None  SaturateOnIntegerOverflow=off  InputSameDT=off
  Multiport Switch2 : MultiPortSwitch  DataPortOrder=Specify indices  DataPortIndices={[4,5],6,3,[1,2]}  DiagnosticForDefault=None  SaturateOnIntegerOverflow=off  InputSameDT=off
  S1 : Outport  VectorParamsAs1DForOutWhenUnconnected=off
  S2 : Outport  Port=2  VectorParamsAs1DForOutWhenUnconnected=off
  S3 : Outport  Port=3  VectorParamsAs1DForOutWhenUnconnected=off
  wires:
  Multiport Switch2/1 -> S3/1
  Multiport Switch1/1 -> S2/1
  0,/1 -> Multiport Switch/5, Multiport Switch1/5, Multiport Switch2/5
  2,0/1 -> Multiport Switch/4, Multiport Switch1/4, Multiport Switch2/4
  1,0/1 -> Multiport Switch/3, Multiport Switch1/3, Multiport Switch2/3
  1,2,0/1 -> Multiport Switch/2, Multiport Switch1/2, Multiport Switch2/2
  Multiport Switch/1 -> S1/1
  sector/1 -> Multiport Switch/1, Multiport Switch1/1, Multiport Switch2/1

== system PID_PMSM_Version_final/Speed controller/SVPWM generator/PWM1/pulsse ==
  Integrator : Integrator
  Pulse Generator : DiscretePulseGenerator  PulseType=Time based  Period=Tsw  PulseWidth=50
  Scope : Scope
  Sum1 : Sum  Inputs=-+|  InputSameDT=on  SaturateOnIntegerOverflow=on  OutDataTypeStr=Inherit: Same as first input
  modulation index2 : Gain  Gain=2  SaturateOnIntegerOverflow=on  OutDataTypeStr=Inherit: Same as input  ParamDataTypeStr=Inherit: Same as input
  pi/1 : Constant  SampleTime=Ts
  pulses : Outport  VectorParamsAs1DForOutWhenUnconnected=off
  wires:
  Pulse Generator/1 -> modulation index2/1
  Integrator/1 -> Scope/1, pulses/1
  modulation index2/1 -> Sum1/2
  Sum1/1 -> Integrator/1
  pi/1/1 -> Sum1/1
